simulink model "AttitudeKalman2"  (Simulink 6.6)
settings: Solver=ode4  StartTime=0.0  StopTime=500  FixedStep=SampleT  RelTol=1e-3
InitFcn:
  | clc
  | Taxi_Var
  | failures
  | insInit
values from neighbouring files (symbols this model uses):
  A1 = 0    [Taxi_Var.m]    (also in Taxi_Var_new.m = 0.007)
  Apolar = 0.0899    [Taxi_Var.m]    (also in Taxi_Var_new.m = 0.057)
  APtsamp = 0.005    [failures.m]    (also in piccolo_init.m = 0.05)
  b0 = [0.01 0.01 0.01]    [insInit.m]
  CD0 = 0.0219    [Taxi_Var.m]    (also in Taxi_Var_new.m = 0.022)
  chord = S/span    (= 0.384036716878)    [Taxi_Var.m]    (also in Taxi_Var_new.m = 0.351341681574)
  CL0 = 0.1857    [Taxi_Var.m]    (also in Taxi_Var_new.m = 0.38)
  CLa = 4.6206    [Taxi_Var.m]    (also in Taxi_Var_new.m = 18.5)
  CLa_dot = 1.93    [Taxi_Var.m]    (also in Taxi_Var_new.m = 2.64)
  Clb = -0.0043    [Taxi_Var.m]    (also in Taxi_Var_new.m = -0.06)
  ClDa = 0.1695    [Taxi_Var.m]    (also in Taxi_Var_new.m)
  CLDe = 0.4032    [Taxi_Var.m]    (also in Taxi_Var_new.m = 0.24)
  CLDf = 0.047    [Taxi_Var.m]    (also in Taxi_Var_new.m = 0.4)
  ClDr = 0.0003    [Taxi_Var.m]    (also in Taxi_Var_new.m = 0.055)
  Clp = -0.4425    [Taxi_Var.m]    (also in Taxi_Var_new.m = -0.88)
  CLq = 8.7465    [Taxi_Var.m]    (also in Taxi_Var_new.m = 7.4)
  Clr = 0.0675    [Taxi_Var.m]    (also in Taxi_Var_new.m = 0.04)
  Cm0 = -0.0902    [Taxi_Var.m]    (also in Taxi_Var_new.m = 0.56)
  Cm0_factor = 0.9    [failures.m]
  Cm0_fail = 0    [failures.m]
  Cma = -1.3995    [Taxi_Var.m]    (also in Taxi_Var_new.m = -1.58)
  CmDe = -0.9493    [Taxi_Var.m]    (also in Taxi_Var_new.m = -41)
  CmDf = -.021    (= -0.021)    [Taxi_Var.m]    (also in Taxi_Var_new.m)
  Cnb = 0.0281    [Taxi_Var.m]    (also in Taxi_Var_new.m = 0.73)
  CnDa = -0.0031    [Taxi_Var.m]    (also in Taxi_Var_new.m = -0.032)
  CnDr = -0.0882    [Taxi_Var.m]    (also in Taxi_Var_new.m = 0.19)
  Cnp = -0.0695    [Taxi_Var.m]    (also in Taxi_Var_new.m = -0.1)
  Cnr = -0.1045    [Taxi_Var.m]    (also in Taxi_Var_new.m = -0.23)
  CYb = -0.1999    [Taxi_Var.m]    (also in Taxi_Var_new.m = -0.98)
  CYDr = 0.0192    [Taxi_Var.m]    (also in Taxi_Var_new.m = 0.066)
  da_failamp = 5    [failures.m]
  da_failbias = -da_failamp/2    (= -2.5)    [failures.m]
  da_failper = 90    [failures.m]
  daL_fail = 0    [failures.m]
  daR_fail = 0    [failures.m]
  dr_fail = 0    [failures.m]
  dr_failamp = 2    [failures.m]
  dr_failbias = -dr_failamp/2    (= -1)    [failures.m]
  dr_failper = 70    [failures.m]
  Euler_0 = [0; 0; 45]'*pi/180    [Taxi_Var.m]    (also in Taxi_Var_new.m = [0 0 45]'*pi/180)
  Gw = zeros(6,6)    [insInit.m]
  H = [eye(3,3) zeros(3,3)]    [insInit.m]
  ISA_g = 9.815    [Taxi_Var.m]    (also in Taxi_Var_new.m)
  Ixx = 3.689084    [Taxi_Var.m]    (also in Taxi_Var_new.m = 3.8)
  Iyy = 7.43789    [Taxi_Var.m]    (also in Taxi_Var_new.m = 9.58)
  Izz = 10.22202    [Taxi_Var.m]    (also in Taxi_Var_new.m = 9.68)
  mass = 22.5    [Taxi_Var.m]    (also in Taxi_Var_new.m = 8.16466266)
  MinThK = 0.075    [Taxi_Var.m]    (also in Taxi_Var_new.m = 0.077)
  P0 = diag([.3 .3 .3  .3 0.75 0.75 0.75 ])    [insInit.m]
  Pos_0 = [0; 0; 1000]'    [Taxi_Var.m]    (also in Taxi_Var_new.m = [0 0 500]')
  PQR_0 = [0; 0; 0]'    [Taxi_Var.m]    (also in Taxi_Var_new.m = [ 0 0 0]'*pi/180)
  Rv = rvv^2*eye(3)    [insInit.m]
  SampleT = 0.005    [failures.m]
  span = 2.3368    [Taxi_Var.m]    (also in Taxi_Var_new.m = 2.795)
  tfailure = 20    [failures.m]
  ThK = 2.18    [Taxi_Var.m]    (also in Taxi_Var_new.m = 2.17)
  Vb_0 = [35; 0; 0]'    [Taxi_Var.m]    (also in Taxi_Var_new.m = [35 0 0]')
undefined symbols (not defined in the file or in its folder): clock, DiscIntNeverNeededParam, Earth, q0, Rw, sigbuilder_block, WGS84
libraries: simulink x25, aerolibconvert2 x8, aerolibactuator x6, dspsigops x5, aerolibutil x5, dspmtrx3 x4, aerolibtransform2 x3, aerolibatmos2 x2, aerolibnav x2, dspinverses x1
(part 2 of 2)

== system AttitudeKalman2/Plant Model/Plant/6-DOF EOM/Get Euler Dot ==
  p,q,r : Inport
  Euler : Inport  Port=2
  Mux1 : Mux  Inputs=[3 3]
  Mux2 : Mux  Inputs=3
  phidot : Fcn  Expr=u[1]+u[2]*sin(u[4])*tan(u[5])+u[3]*cos(u[4])*tan(u[5])
  psidot : Fcn  Expr=u[2]*sin(u[4])/cos(u[5])+u[3]*cos(u[4])/cos(u[5])
  thetadot : Fcn  Expr=u[2]*cos(u[4])-u[3]*sin(u[4])
  Euler_dot : Outport
  wires:
  Mux2/1 -> Euler_dot/1
  phidot/1 -> Mux2/1
  thetadot/1 -> Mux2/2
  psidot/1 -> Mux2/3
  Mux1/1 -> thetadot/1, phidot/1, psidot/1
  p,q,r/1 -> Mux1/1
  Euler/1 -> Mux1/2

== system AttitudeKalman2/Plant Model/Plant/6-DOF EOM/RB2LTP ==
  Euler : Inport
  11 : Fcn  Expr=cos(u[3])*cos(u[2])
  12 : Fcn  Expr=sin(u[3])*cos(u[2])
  13 : Fcn  Expr=-sin(u[2])
  21 : Fcn  Expr=cos(u[3])*sin(u[2])*sin(u[1])-sin(u[3])*cos(u[1])
  22 : Fcn  Expr=sin(u[3])*sin(u[2])*sin(u[1])+cos(u[3])*cos(u[1])
  23 : Fcn  Expr=cos(u[2])*sin(u[1])
  31 : Fcn  Expr=cos(u[3])*sin(u[2])*cos(u[1])+sin(u[3])*sin(u[1])
  32 : Fcn  Expr=sin(u[3])*sin(u[2])*cos(u[1])-cos(u[3])*sin(u[1])
  33 : Fcn  Expr=cos(u[2])*cos(u[1])
  Mux2 : Mux  Inputs=9
  Reshape : Reshape  OutputDimensionality=Customize  OutputDimensions=[3,3]
  Rot : Outport
  wires:
  33/1 -> Mux2/9
  32/1 -> Mux2/8
  31/1 -> Mux2/7
  23/1 -> Mux2/6
  22/1 -> Mux2/5
  21/1 -> Mux2/4
  13/1 -> Mux2/3
  12/1 -> Mux2/2
  11/1 -> Mux2/1
  Mux2/1 -> Reshape/1
  Euler/1 -> 11/1, 33/1, 32/1, 31/1, 23/1, 22/1, 21/1, 13/1, 12/1
  Reshape/1 -> Rot/1

== system AttitudeKalman2/Plant Model/Plant/6-DOF EOM/[V1,2,3,W1,2,3] ==
  note: V*dot =Inv(A){[F ; M] - SigmaAV*}
  "[F ; M]" : Inport
  Euler : Inport  Port=2
  V* : Inport  Port=3  PortDimensions=6
  A = [M ; J] : Subsystem
  Acc_meas : Product  Inputs=/*  Multiplication=Matrix(*)  SaturateOnIntegerOverflow=on  InputSameDT=on
  Demux : Demux  Outputs=[3;3]
  Get Grav Force in Body : Subsystem
  Gravitational Acc : Constant  Value=[0 0 -ISA_g]  VectorParams1D=off
  Selector3 : Selector  IndexOptions=Index vector (dialog)  Indices=1:3  OutputSizes=1  InputPortWidth=6
  Sigma : Subsystem
  Sigma*A : Product  Multiplication=Matrix(*)  SaturateOnIntegerOverflow=on  InputSameDT=on
  Sigma*A*V* : Product  Multiplication=Matrix(*)  SaturateOnIntegerOverflow=on  InputSameDT=on
  Sum1 : Sum  Inputs=+-|  SaturateOnIntegerOverflow=on  InputSameDT=on
  Sum2 : Sum  Inputs=++|  SaturateOnIntegerOverflow=on  InputSameDT=on
  Terminator1 : Terminator
  "V*dot " : Product  Inputs=/*  Multiplication=Matrix(*)  SaturateOnIntegerOverflow=on  InputSameDT=on
  "Acc_meas " : Outport
  V*dot : Outport  Port=2
  wires:
  Sum1/1 -> "V*dot "/2
  A = [M ; J]/1(A Matrix) -> Sigma*A/2, "V*dot "/1, Acc_meas/1
  Demux/1 -> Terminator1/1
  Sigma/1(Sigma) -> Sigma*A/1
  "[F ; M]"/1 -> Sum1/1, Acc_meas/2
  Sigma*A*V*/1 -> Sum1/2
  Demux/2 -> Sigma/1(pqr)
  V*/1 -> Sigma*A*V*/2, Demux/1
  "V*dot "/1 -> V*dot/1
  Sigma*A/1 -> Sigma*A*V*/1
  Acc_meas/1 -> Selector3/1
  Gravitational Acc/1 -> Get Grav Force in Body/2(Grav Force)
  Euler/1 -> Get Grav Force in Body/1(Euler)
  Selector3/1 -> Sum2/2
  Get Grav Force in Body/1(Grav Force (Body)) -> Sum2/1
  Sum2/1 -> "Acc_meas "/1

== system AttitudeKalman2/Plant Model/Plant/Engine Model/Get To1 ==
  dt : Inport
  Divide : Product  Inputs=3  OutScaling=2^-10
  Math Function : Math  Operator=pow  SaturateOnIntegerOverflow=on
  Math Function1 : Math  Operator=pow  SaturateOnIntegerOverflow=on
  MaxRPM : Gain  Gain=7200  SaturateOnIntegerOverflow=on
  Min RPM : Constant  Value=2000
  Min Th K : Constant  Value=MinThK
  Prop Diameter (in) : Constant  Value=17
  Prop Diameter (in)1 : Constant  Value=2
  Prop Diameter (in)2 : Constant  Value=4
  Saturation : Saturate  UpperLimit=1.0  LowerLimit=0.2
  Sum : Sum  Inputs=|++
  Sum1 : Sum  Inputs=|++
  TFact : simulink/Math Operations/Slider Gain  SystemSampleTime=-1  low=0  gain=0.2  high=1
  Th K : Gain  Gain=ThK  SaturateOnIntegerOverflow=on
  To Constant : Constant  Value=2.83e-12
  RPM : Outport
  To : Outport  Port=2
  wires:
  Min Th K/1 -> Sum1/2
  Sum1/1 -> MaxRPM/1
  dt/1 -> Saturation/1
  Th K/1 -> Sum1/1
  MaxRPM/1 -> Sum/1
  Min RPM/1 -> Sum/2
  Sum/1 -> RPM/1, Math Function/1
  TFact/1 -> To/1
  Divide/1 -> TFact/1
  To Constant/1 -> Divide/3
  Math Function1/1 -> Divide/2
  Math Function/1 -> Divide/1
  Prop Diameter (in)/1 -> Math Function1/1
  Prop Diameter (in)2/1 -> Math Function1/2
  Prop Diameter (in)1/1 -> Math Function/2
  Saturation/1 -> Th K/1

== system AttitudeKalman2/Plant Model/Plant/Forces and Moments/Alpha/Beta ==
  "Vx, Vy, Vz (Body)" : Inport
  Rho : Inport  Port=2
  Constant : Constant  Value=0.5  VectorParams1D=off
  Math Function : Math  Operator=sqrt  SaturateOnIntegerOverflow=on
  Product : Product  Inputs=5  SaturateOnIntegerOverflow=on
  R2D1 : Gain  Gain=180/pi  SaturateOnIntegerOverflow=on
  R2D2 : Gain  Gain=180/pi  SaturateOnIntegerOverflow=on
  Scope : Scope
      settings: YMin=-2.5  YMax=2  SaveName=ScopeData6
  Scope1 : Scope
      settings: YMin=-1.5  YMax=1.5  SaveName=ScopeData8
  V^2 : Fcn  Expr=(u(1)^2+u(2)^2+u(3)^2)
  "[-15; 15 ]" : Saturate  UpperLimit=15  LowerLimit=-15
  "[-15;15]" : Saturate  UpperLimit=15  LowerLimit=-15
  aoa : Trigonometry  Operator=asin
  beta : Trigonometry  Operator=atan
  sin(aoa) : Fcn  Expr=u(3)/sqrt(u(1)^2+u(3)^2)
  span : Constant  Value=span  VectorParams1D=off
  span1 : Constant  Value=chord  VectorParams1D=off
  tan(beta) : Fcn  Expr=u(2)/sqrt(u(1)^2+u(3)^2)
  "alpha, deg" : Outport
  "beta, deg" : Outport  Port=2
  qS : Outport  Port=3
  Speed : Outport  Port=4
  wires:
  "Vx, Vy, Vz (Body)"/1 -> sin(aoa)/1, tan(beta)/1, V^2/1
  tan(beta)/1 -> beta/1
  beta/1 -> R2D1/1
  V^2/1 -> Product/1, Math Function/1
  Rho/1 -> Product/2
  Constant/1 -> Product/3
  Product/1 -> qS/1
  span/1 -> Product/4
  span1/1 -> Product/5
  R2D1/1 -> "[-15; 15 ]"/1  "beta"
  aoa/1 -> R2D2/1
  R2D2/1 -> "[-15;15]"/1  "aoa"
  sin(aoa)/1 -> aoa/1
  Math Function/1 -> Speed/1
  "[-15;15]"/1 -> "alpha, deg"/1, Scope1/1
  "[-15; 15 ]"/1 -> "beta, deg"/1, Scope/1

== system AttitudeKalman2/Plant Model/Plant/Forces and Moments/Body Frame F & M ==
  "Alpha, deg" : Inport
  "Beta, deg" : Inport  Port=2
  qs : Inport  Port=3
  Airspeed : Inport  Port=4
  "de, deg" : Inport  Port=5
  "dr, deg" : Inport  Port=6
  "df, deg" : Inport  Port=7
  "da_L, deg" : Inport  Port=8
  "da_R, deg" : Inport  Port=9
  p,q,r : Inport  Port=10
  Bus Creator : BusCreator  Inputs=2
  Transfer to body frame : Subsystem
  Wind frame F& M : Subsystem
  F_b : Outport
  M_b : Outport  Port=2
  wires:
  "Alpha, deg"/1 -> Wind frame F& M/1("alpha, deg"), Bus Creator/1
  "Beta, deg"/1 -> Wind frame F& M/2("beta, deg"), Bus Creator/2
  "dr, deg"/1 -> Wind frame F& M/4("dr, deg")
  "da_L, deg"/1 -> Wind frame F& M/9("da_L, deg")
  "de, deg"/1 -> Wind frame F& M/3("de, deg")
  Wind frame F& M/1(F&M wind frame) -> Transfer to body frame/1(Wind frame  F&M)
  Bus Creator/1 -> Transfer to body frame/2("aoa/beta, deg")  "aoa/beta, deg"
  Transfer to body frame/1(F_b) -> F_b/1
  Transfer to body frame/2(M_b) -> M_b/1
  "df, deg"/1 -> Wind frame F& M/5("df, deg")
  qs/1 -> Wind frame F& M/6(qS)
  p,q,r/1 -> Wind frame F& M/7(p,q,r)
  Airspeed/1 -> Wind frame F& M/8(Airpseed)
  "da_R, deg"/1 -> Wind frame F& M/10("da_R, deg")

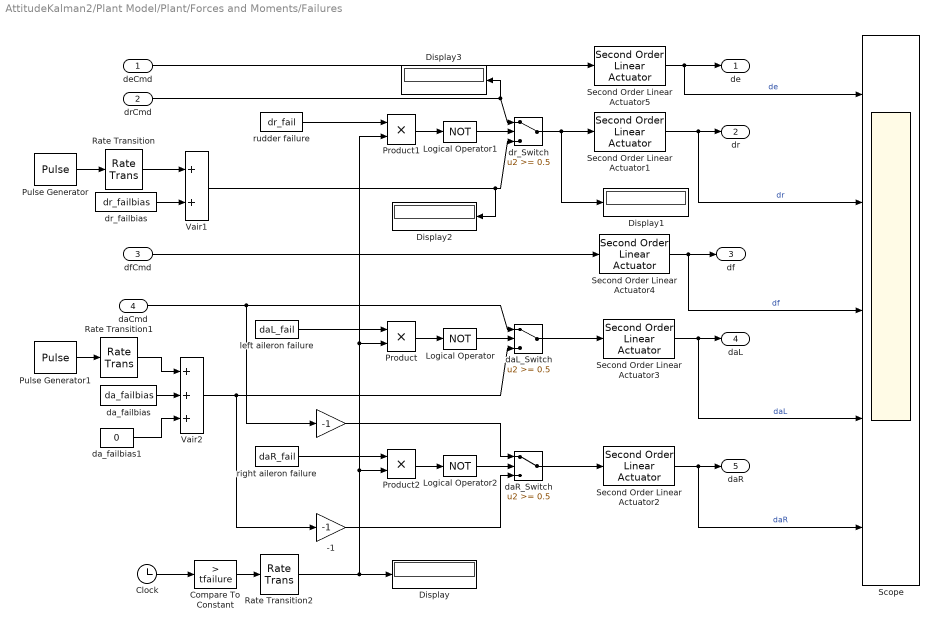
== system AttitudeKalman2/Plant Model/Plant/Forces and Moments/Failures ==
  deCmd : Inport
  drCmd : Inport  Port=2
  dfCmd : Inport  Port=3
  daCmd : Inport  Port=4
  " " : Gain  Gain=-1  SaturateOnIntegerOverflow=on
  "-1 " : Gain  Gain=-1  SaturateOnIntegerOverflow=on
  Clock : Clock
      settings: Decimation=10
  Compare To Constant : simulink/Logic and Bit Operations/Compare To Constant  SystemSampleTime=-1  relop=>  const=tfailure  LogicOutDataTypeMode=uint8  ZeroCross=off
  Display{,1..3} (4 alike) : Display
  Logical Operator : Logic  Operator=NOT  AllPortsSameDT=off  OutDataTypeMode=Boolean
  Logical Operator1 : Logic  Operator=NOT  AllPortsSameDT=off  OutDataTypeMode=Boolean
  Logical Operator2 : Logic  Operator=NOT  AllPortsSameDT=off  OutDataTypeMode=Boolean
  Product : Product  RndMeth=Zero
  Product1 : Product  RndMeth=Zero
  Product2 : Product  RndMeth=Zero
  Pulse Generator : DiscretePulseGenerator  PulseType=Time based  Amplitude=dr_failamp  Period=dr_failper  PulseWidth=50
  Pulse Generator1 : DiscretePulseGenerator  PulseType=Time based  Amplitude=da_failamp  Period=da_failper  PulseWidth=50
  Rate Transition : RateTransition  OutPortSampleTime=APtsamp
  Rate Transition1 : RateTransition  OutPortSampleTime=APtsamp
  Rate Transition2 : RateTransition  OutPortSampleTime=APtsamp
  Scope : Scope  NumInputPorts=5
      settings: YMin=-5~-5~-5~-5~-5  YMax=5~5~5~5~5  SaveName=ScopeData5
  Second Order Linear Actuator{1..5} (5 alike) : aerolibactuator/Second Order Linear Actuator  SystemSampleTime=-1  wn_fin=60  z_fin=0.7  fin_act_0=0
  Vair1 : Sum  SaturateOnIntegerOverflow=on  InputSameDT=on
  Vair2 : Sum  Inputs=+++  SaturateOnIntegerOverflow=on  InputSameDT=on
  daL_Switch : Switch  Threshold=0.5
  daR_Switch : Switch  Threshold=0.5
  da_failbias : Constant  Value=da_failbias  SampleTime=APtsamp
  da_failbias1 : Constant  Value=0  SampleTime=APtsamp
  dr_Switch : Switch  Threshold=0.5
  dr_failbias : Constant  Value=dr_failbias  SampleTime=APtsamp
  left aileron failure : Constant  Value=daL_fail  SampleTime=APtsamp
  right aileron failure : Constant  Value=daR_fail  SampleTime=APtsamp
  rudder failure : Constant  Value=dr_fail  SampleTime=APtsamp
  de : Outport
  dr : Outport  Port=2
  df : Outport  Port=3
  daL : Outport  Port=4
  daR : Outport  Port=5
  wires:
  Pulse Generator/1 -> Rate Transition/1
  dr_failbias/1 -> Vair1/2
  deCmd/1 -> Second Order Linear Actuator5/1
  dr_Switch/1 -> Second Order Linear Actuator1/1, Display1/1
  rudder failure/1 -> Product1/1
  drCmd/1 -> dr_Switch/1, Display3/1
  Vair1/1 -> dr_Switch/3, Display2/1
  dfCmd/1 -> Second Order Linear Actuator4/1
  Pulse Generator1/1 -> Rate Transition1/1
  da_failbias/1 -> Vair2/2
  left aileron failure/1 -> Product/1
  daCmd/1 -> daL_Switch/1, " "/1
  Vair2/1 -> daL_Switch/3, "-1 "/1
  daL_Switch/1 -> Second Order Linear Actuator3/1
  right aileron failure/1 -> Product2/1
  daR_Switch/1 -> Second Order Linear Actuator2/1
  " "/1 -> daR_Switch/1
  "-1 "/1 -> daR_Switch/3
  Second Order Linear Actuator1/1 -> dr/1, Scope/2  "dr"
  Second Order Linear Actuator3/1 -> daL/1, Scope/4  "daL"
  Second Order Linear Actuator2/1 -> daR/1, Scope/5  "daR"
  Second Order Linear Actuator5/1 -> de/1, Scope/1  "de"
  Second Order Linear Actuator4/1 -> df/1, Scope/3  "df"
  Clock/1 -> Compare To Constant/1
  Product/1 -> Logical Operator/1
  Product1/1 -> Logical Operator1/1
  Product2/1 -> Logical Operator2/1
  Compare To Constant/1 -> Rate Transition2/1
  Logical Operator1/1 -> dr_Switch/2
  Logical Operator/1 -> daL_Switch/2
  Logical Operator2/1 -> daR_Switch/2
  da_failbias1/1 -> Vair2/3
  Rate Transition/1 -> Vair1/1
  Rate Transition1/1 -> Vair2/1
  Rate Transition2/1 -> Product2/2, Product/2, Product1/2, Display/1

== system AttitudeKalman2/Plant Model/Plant/Forces and Moments/Get Grav Force in Body ==
  Euler : Inport
  Grav Force : Inport  Port=2
  Math Function : Math  Operator=transpose  SaturateOnIntegerOverflow=on
  Product1 : Product  Multiplication=Matrix(*)  SaturateOnIntegerOverflow=on  InputSameDT=on
  Rb2u : Subsystem
  Reshape : Reshape  OutputDimensionality=Column vector (2-D)
  Grav Force (Body) : Outport
  wires:
  Rb2u/1(DCM) -> Math Function/1
  Euler/1 -> Rb2u/1(phi theta psi)
  Product1/1 -> Grav Force (Body)/1
  Math Function/1 -> Product1/1
  Grav Force/1 -> Reshape/1
  Reshape/1 -> Product1/2

== system AttitudeKalman2/Plant Model/Plant/Forces and Moments/NED(u)2b ==
  V w : Inport
  Euler : Inport  Port=2
  RB2LTP : Subsystem
  RL2B * Vw : Product  Multiplication=Matrix(*)  SaturateOnIntegerOverflow=on  InputSameDT=on
  RLTP2B : Math  Operator=transpose  SaturateOnIntegerOverflow=on
  Reshape1 : Reshape  OutputDimensionality=Row vector (2-D)
  Vb Corr : Outport
  wires:
  RL2B * Vw/1 -> Reshape1/1
  Euler/1 -> RB2LTP/1(Euler)
  RB2LTP/1(RB2L) -> RLTP2B/1
  RLTP2B/1 -> RL2B * Vw/1
  V w/1 -> RL2B * Vw/2
  Reshape1/1 -> Vb Corr/1

== system AttitudeKalman2/Get GPS in LTP/Geod2LTP2/ECEF2LTP (UEN)/From Body to Universal1/Rotation Matrix from Long//Lat ==
  note: Calculate Coefficients of DCM Row-Wise
  long lat : Inport
  11 : Fcn  Expr=cos(u[1])*cos(u[2])
  12 : Fcn  Expr=sin(u[1])*cos(u[2])
  13 : Fcn  Expr=sin(u[2])
  21 : Fcn  Expr=-sin(u[1])
  22 : Fcn  Expr=cos(u[1])
  23 : Fcn  Expr=0
  31 : Fcn  Expr=-sin(u[2])*cos(u[1])
  32 : Fcn  Expr=-sin(u[1])*sin(u[2])
  33 : Fcn  Expr=cos(u[2])
  Mux2 : Mux  Inputs=9
  DCM : Outport  InitialOutput=0
  wires:
  33/1 -> Mux2/9
  23/1 -> Mux2/8
  13/1 -> Mux2/7
  32/1 -> Mux2/6
  22/1 -> Mux2/5
  12/1 -> Mux2/4
  31/1 -> Mux2/3
  21/1 -> Mux2/2
  11/1 -> Mux2/1
  Mux2/1 -> DCM/1
  long lat/1 -> 11/1, 33/1, 23/1, 13/1, 32/1, 22/1, 12/1, 31/1, 21/1

== system AttitudeKalman2/Plant Model/Plant/6-DOF EOM/[V1,2,3,W1,2,3]/A = [M ; J] ==
  Constant1 : Constant  Value=zeros(3,3)
  Constant4 : Constant  Value=0
  Display : Display
  Display1 : Display
  Display2 : Display
  Ixx : Constant  Value=Ixx  VectorParams1D=off
  Iyy : Constant  Value=Iyy  VectorParams1D=off
  Izz : Constant  Value=Izz  VectorParams1D=off
  Matrix Concatenation : Concatenate  Mode=Multidimensional array
  Matrix Concatenation1 : Concatenate  Mode=Multidimensional array
  Matrix Concatenation2 : Concatenate  Mode=Multidimensional array  ConcatenateDimension=2
  Mux : Mux  Inputs=9
  Mux1 : Mux  Inputs=9
  Reshape : Reshape  OutputDimensionality=Customize  OutputDimensions=[3,3]
  Reshape1 : Reshape  OutputDimensionality=Customize  OutputDimensions=[3,3]
  mass : Constant  Value=mass  VectorParams1D=off
  A Matrix : Outport
  wires:
  Constant1/1 -> Matrix Concatenation1/1, Matrix Concatenation/2
  Reshape/1 -> Matrix Concatenation/1
  Reshape1/1 -> Matrix Concatenation1/2
  Matrix Concatenation2/1 -> Display2/1, A Matrix/1
  Matrix Concatenation1/1 -> Display1/1, Matrix Concatenation2/2
  Matrix Concatenation/1 -> Display/1, Matrix Concatenation2/1
  Mux/1 -> Reshape1/1
  Mux1/1 -> Reshape/1
  mass/1 -> Mux1/9, Mux1/5, Mux1/1
  Constant4/1 -> Mux1/2, Mux1/3, Mux1/4, Mux1/6, Mux1/7, Mux1/8, Mux/2, Mux/3, Mux/4, Mux/6, Mux/7, Mux/8
  Iyy/1 -> Mux/5
  Izz/1 -> Mux/9
  Ixx/1 -> Mux/1

== system AttitudeKalman2/Plant Model/Plant/6-DOF EOM/[V1,2,3,W1,2,3]/Get Grav Force in Body ==
  Euler : Inport
  Grav Force : Inport  Port=2
  Math Function : Math  Operator=transpose  SaturateOnIntegerOverflow=on
  Product1 : Product  Multiplication=Matrix(*)  SaturateOnIntegerOverflow=on  InputSameDT=on
  Rb2u : Subsystem
  Reshape : Reshape  OutputDimensionality=Column vector (2-D)
  Grav Force (Body) : Outport
  wires:
  Reshape/1 -> Product1/2
  Grav Force/1 -> Reshape/1
  Math Function/1 -> Product1/1
  Product1/1 -> Grav Force (Body)/1
  Euler/1 -> Rb2u/1(phi theta psi)
  Rb2u/1(DCM) -> Math Function/1

== system AttitudeKalman2/Plant Model/Plant/6-DOF EOM/[V1,2,3,W1,2,3]/Sigma ==
  note: S(pqr)
  pqr : Inport
  Gain : Gain  Gain=[0 0 0;0 0 -1; 0 1 0]  Multiplication=Matrix(K*u)  SaturateOnIntegerOverflow=on
  Gain1 : Gain  Gain=[0 0 1;0 0 0; -1 0 0]  Multiplication=Matrix(K*u)  SaturateOnIntegerOverflow=on
  Gain2 : Gain  Gain="[0 -1 0;1 0 0;  0 0 0]"  Multiplication=Matrix(K*u)  SaturateOnIntegerOverflow=on
  Gain3 : Gain  Gain=0  SaturateOnIntegerOverflow=on
  Math Function : Math  Operator=transpose  SaturateOnIntegerOverflow=on
  Matrix Concatenation : Concatenate  Mode=Multidimensional array  ConcatenateDimension=2
  Matrix Concatenation1 : Concatenate  Mode=Multidimensional array  ConcatenateDimension=2
  Matrix Concatenation2 : Concatenate  Mode=Multidimensional array
  Mux : Mux  Inputs=3
  Reshape : Reshape  OutputDimensionality=Customize  OutputDimensions=[3,3]
  Sigma : Outport
  wires:
  pqr/1 -> Gain1/1, Gain2/1, Gain/1
  Matrix Concatenation2/1 -> Sigma/1
  Matrix Concatenation1/1 -> Matrix Concatenation2/2
  Matrix Concatenation/1 -> Matrix Concatenation2/1
  Gain3/1 -> Matrix Concatenation1/1, Matrix Concatenation/2
  Math Function/1 -> Matrix Concatenation1/2, Matrix Concatenation/1, Gain3/1
  Reshape/1 -> Math Function/1
  Gain2/1 -> Mux/3
  Gain1/1 -> Mux/2
  Gain/1 -> Mux/1
  Mux/1 -> Reshape/1

== system AttitudeKalman2/Plant Model/Plant/Forces and Moments/Body Frame F & M/Transfer to body frame ==
  Wind frame  F&M : Inport
  "aoa/beta, deg" : Inport  Port=2
  D2R : Gain  Gain=pi/180  SaturateOnIntegerOverflow=on
  Forces : Selector  IndexOptions=Index vector (dialog)  Indices=[1 2 3]  OutputSizes=[(-2)]  InputPortWidth=6
  Moments : Selector  IndexOptions=Index vector (dialog)  Indices=[4 5 6]  OutputSizes=[(-2)]  InputPortWidth=6
  Ra2b1 : Subsystem
  Ra2b22 : Subsystem
  Scope : Scope
      settings: YMin=-450  YMax=200  SaveName=ScopeData11
  F_b : Outport
  M_b : Outport  Port=2
  wires:
  Ra2b1/1(body frame) -> F_b/1, Scope/1  "Fb"
  Ra2b22/1(body frame) -> M_b/1  "Mb"
  "aoa/beta, deg"/1 -> D2R/1
  Forces/1 -> Ra2b1/1(wind frame)
  Wind frame  F&M/1 -> Forces/1, Moments/1
  Moments/1 -> Ra2b22/2(wind frame)
  D2R/1 -> Ra2b1/2(aoa/beta), Ra2b22/1(aoa/beta)

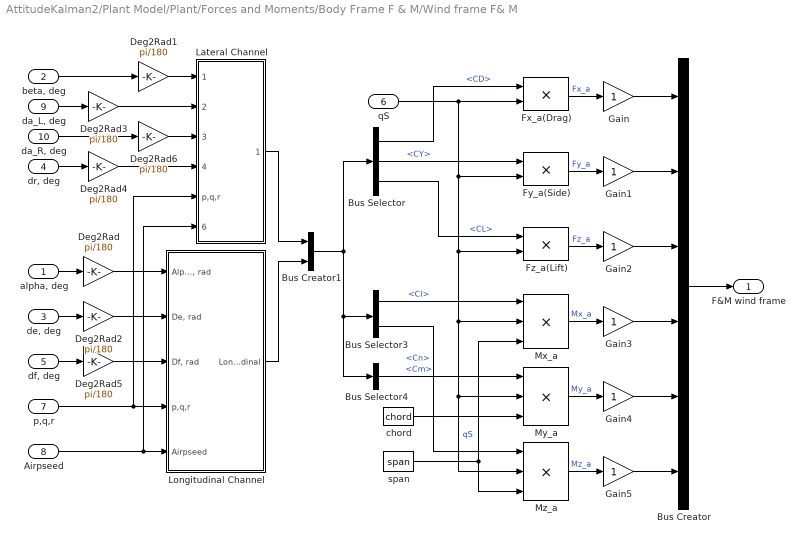
== system AttitudeKalman2/Plant Model/Plant/Forces and Moments/Body Frame F & M/Wind frame F& M ==
  "alpha, deg" : Inport
  "beta, deg" : Inport  Port=2
  "de, deg" : Inport  Port=3
  "dr, deg" : Inport  Port=4
  "df, deg" : Inport  Port=5
  qS : Inport  Port=6
  p,q,r : Inport  Port=7
  Airpseed : Inport  Port=8
  "da_L, deg" : Inport  Port=9
  "da_R, deg" : Inport  Port=10
  Bus Creator : BusCreator  Inputs=6
  Bus Creator1 : BusCreator  Inputs=2
  Bus Selector : BusSelector  OutputSignals=signal2.CD,signal1.CY,signal2.CL
  Bus Selector3 : BusSelector  OutputSignals=signal1.Cl,signal1.Cn
  Bus Selector4 : BusSelector  OutputSignals=signal2.Cm
  Deg2Rad{,1..6} (7 alike) : Gain  Gain=pi/180  SaturateOnIntegerOverflow=on
  Fx_a(Drag) : Product  Inputs=**  SaturateOnIntegerOverflow=on
  Fy_a(Side) : Product  SaturateOnIntegerOverflow=on
  Fz_a(Lift) : Product  SaturateOnIntegerOverflow=on
  Gain{,1..5} (6 alike) : Gain  SaturateOnIntegerOverflow=on
  Lateral Channel : Subsystem
  Longitudinal Channel : Subsystem
  Mx_a : Product  Inputs=3  SaturateOnIntegerOverflow=on
  My_a : Product  Inputs=3  SaturateOnIntegerOverflow=on
  Mz_a : Product  Inputs=3  SaturateOnIntegerOverflow=on
  chord : Constant  Value=chord  VectorParams1D=off
  span : Constant  Value=span  VectorParams1D=off
  F&M wind frame : Outport
  wires:
  Bus Selector/1 -> Fx_a(Drag)/1  "<CD>"
  Fx_a(Drag)/1 -> Gain/1  "Fx_a"
  Fy_a(Side)/1 -> Gain1/1  "Fy_a"
  Fz_a(Lift)/1 -> Gain2/1  "Fz_a"
  Bus Selector3/1 -> Mx_a/1  "<Cl>"
  Mx_a/1 -> Gain3/1  "Mx_a"
  Bus Selector4/1 -> My_a/1  "<Cm>"
  Mz_a/1 -> Gain5/1  "Mz_a"
  qS/1 -> Fx_a(Drag)/2, Fy_a(Side)/2, Fz_a(Lift)/2, Mx_a/2, My_a/2, Mz_a/2  "qS"
  span/1 -> Mx_a/3, Mz_a/3
  chord/1 -> My_a/3
  Bus Selector/2 -> Fy_a(Side)/1  "<CY>"
  Bus Selector/3 -> Fz_a(Lift)/1  "<CL>"
  Bus Selector3/2 -> Mz_a/1  "<Cn>"
  Bus Creator/1 -> F&M wind frame/1
  My_a/1 -> Gain4/1  "My_a"
  Bus Creator1/1 -> Bus Selector/1, Bus Selector3/1, Bus Selector4/1
  Longitudinal Channel/1(Longitudinal) -> Bus Creator1/2
  "alpha, deg"/1 -> Deg2Rad/1
  "beta, deg"/1 -> Deg2Rad1/1
  "de, deg"/1 -> Deg2Rad2/1
  "da_L, deg"/1 -> Deg2Rad3/1
  "dr, deg"/1 -> Deg2Rad4/1
  Deg2Rad1/1 -> Lateral Channel/1("beta, rad")
  Deg2Rad4/1 -> Lateral Channel/4("Dr, rad")
  Deg2Rad/1 -> Longitudinal Channel/1("Alpha, rad")
  Deg2Rad2/1 -> Longitudinal Channel/2("De, rad")
  Gain/1 -> Bus Creator/1
  Gain1/1 -> Bus Creator/2
  Gain2/1 -> Bus Creator/3
  Gain3/1 -> Bus Creator/4
  Gain4/1 -> Bus Creator/5
  Gain5/1 -> Bus Creator/6
  "df, deg"/1 -> Deg2Rad5/1
  Deg2Rad5/1 -> Longitudinal Channel/3("Df, rad")
  Lateral Channel/1(Lateral) -> Bus Creator1/1
  p,q,r/1 -> Lateral Channel/5(p,q,r), Longitudinal Channel/4(p,q,r)
  Airpseed/1 -> Lateral Channel/6(Airspeed), Longitudinal Channel/5(Airpseed)
  Deg2Rad3/1 -> Lateral Channel/2("Da L, rad")
  Deg2Rad6/1 -> Lateral Channel/3("Da R, rad")
  "da_R, deg"/1 -> Deg2Rad6/1

== system AttitudeKalman2/Plant Model/Plant/Forces and Moments/Get Grav Force in Body/Rb2u ==
  phi theta psi : Inport
  11 : Fcn  Expr=cos(u[3])*cos(u[2])
  12 : Fcn  Expr=sin(u[3])*cos(u[2])
  13 : Fcn  Expr=-sin(u[2])
  21 : Fcn  Expr=cos(u[3])*sin(u[2])*sin(u[1])-sin(u[3])*cos(u[1])
  22 : Fcn  Expr=sin(u[3])*sin(u[2])*sin(u[1])+cos(u[3])*cos(u[1])
  23 : Fcn  Expr=cos(u[2])*sin(u[1])
  31 : Fcn  Expr=cos(u[3])*sin(u[2])*cos(u[1])+sin(u[3])*sin(u[1])
  32 : Fcn  Expr=sin(u[3])*sin(u[2])*cos(u[1])-cos(u[3])*sin(u[1])
  33 : Fcn  Expr=cos(u[2])*cos(u[1])
  Mux2 : Mux  Inputs=9
  Reshape : Reshape  OutputDimensionality=Customize  OutputDimensions=[3,3]
  DCM : Outport  InitialOutput=0
  wires:
  Reshape/1 -> DCM/1
  phi theta psi/1 -> 12/1, 13/1, 21/1, 22/1, 23/1, 31/1, 32/1, 33/1, 11/1
  Mux2/1 -> Reshape/1
  11/1 -> Mux2/1
  12/1 -> Mux2/2
  13/1 -> Mux2/3
  21/1 -> Mux2/4
  22/1 -> Mux2/5
  23/1 -> Mux2/6
  31/1 -> Mux2/7
  32/1 -> Mux2/8
  33/1 -> Mux2/9

== system AttitudeKalman2/Plant Model/Plant/Forces and Moments/NED(u)2b/RB2LTP ==
  Euler : Inport
  11 : Fcn  Expr=cos(u[3])*cos(u[2])
  12 : Fcn  Expr=sin(u[3])*cos(u[2])
  13 : Fcn  Expr=-sin(u[2])
  21 : Fcn  Expr=cos(u[3])*sin(u[2])*sin(u[1])-sin(u[3])*cos(u[1])
  22 : Fcn  Expr=sin(u[3])*sin(u[2])*sin(u[1])+cos(u[3])*cos(u[1])
  23 : Fcn  Expr=cos(u[2])*sin(u[1])
  31 : Fcn  Expr=cos(u[3])*sin(u[2])*cos(u[1])+sin(u[3])*sin(u[1])
  32 : Fcn  Expr=sin(u[3])*sin(u[2])*cos(u[1])-cos(u[3])*sin(u[1])
  33 : Fcn  Expr=cos(u[2])*cos(u[1])
  Mux2 : Mux  Inputs=9
  Reshape : Reshape  OutputDimensionality=Customize  OutputDimensions=[3,3]
  RB2L : Outport  InitialOutput=0
  wires:
  33/1 -> Mux2/9
  32/1 -> Mux2/8
  31/1 -> Mux2/7
  23/1 -> Mux2/6
  22/1 -> Mux2/5
  21/1 -> Mux2/4
  13/1 -> Mux2/3
  12/1 -> Mux2/2
  11/1 -> Mux2/1
  Mux2/1 -> Reshape/1
  Euler/1 -> 11/1, 33/1, 32/1, 31/1, 23/1, 22/1, 21/1, 13/1, 12/1
  Reshape/1 -> RB2L/1

== system AttitudeKalman2/Plant Model/Plant/6-DOF EOM/[V1,2,3,W1,2,3]/Get Grav Force in Body/Rb2u ==
  phi theta psi : Inport
  11 : Fcn  Expr=cos(u[3])*cos(u[2])
  12 : Fcn  Expr=sin(u[3])*cos(u[2])
  13 : Fcn  Expr=-sin(u[2])
  21 : Fcn  Expr=cos(u[3])*sin(u[2])*sin(u[1])-sin(u[3])*cos(u[1])
  22 : Fcn  Expr=sin(u[3])*sin(u[2])*sin(u[1])+cos(u[3])*cos(u[1])
  23 : Fcn  Expr=cos(u[2])*sin(u[1])
  31 : Fcn  Expr=cos(u[3])*sin(u[2])*cos(u[1])+sin(u[3])*sin(u[1])
  32 : Fcn  Expr=sin(u[3])*sin(u[2])*cos(u[1])-cos(u[3])*sin(u[1])
  33 : Fcn  Expr=cos(u[2])*cos(u[1])
  Mux2 : Mux  Inputs=9
  Reshape : Reshape  OutputDimensionality=Customize  OutputDimensions=[3,3]
  DCM : Outport  InitialOutput=0
  wires:
  33/1 -> Mux2/9
  32/1 -> Mux2/8
  31/1 -> Mux2/7
  23/1 -> Mux2/6
  22/1 -> Mux2/5
  21/1 -> Mux2/4
  13/1 -> Mux2/3
  12/1 -> Mux2/2
  11/1 -> Mux2/1
  Mux2/1 -> Reshape/1
  phi theta psi/1 -> 11/1, 33/1, 32/1, 31/1, 23/1, 22/1, 21/1, 13/1, 12/1
  Reshape/1 -> DCM/1

== system AttitudeKalman2/Plant Model/Plant/Forces and Moments/Body Frame F & M/Transfer to body frame/Ra2b1 ==
  wind frame : Inport
  aoa/beta : Inport  Port=2
  Product2 : Product  Multiplication=Matrix(*)  SaturateOnIntegerOverflow=on
  RB2W : Subsystem
  RW2B : Math  Operator=transpose  SaturateOnIntegerOverflow=on
  Reshape : Reshape  OutputDimensionality=Column vector (2-D)
  body frame : Outport
  wires:
  RB2W/1(Rw2b) -> RW2B/1
  aoa/beta/1 -> RB2W/1(aoa beta)
  Product2/1 -> body frame/1
  wind frame/1 -> Reshape/1
  Reshape/1 -> Product2/2
  RW2B/1 -> Product2/1

== system AttitudeKalman2/Plant Model/Plant/Forces and Moments/Body Frame F & M/Transfer to body frame/Ra2b22 ==
  aoa/beta : Inport
  wind frame : Inport  Port=2
  Product2 : Product  Multiplication=Matrix(*)  SaturateOnIntegerOverflow=on
  RB2W : Subsystem
  RW2B : Math  Operator=transpose  SaturateOnIntegerOverflow=on
  Reshape : Reshape  OutputDimensionality=Column vector (2-D)
  body frame : Outport
  wires:
  Reshape/1 -> Product2/2
  wind frame/1 -> Reshape/1
  Product2/1 -> body frame/1
  aoa/beta/1 -> RB2W/1(aoa beta)
  RB2W/1(Rw2b) -> RW2B/1
  RW2B/1 -> Product2/1

== system AttitudeKalman2/Plant Model/Plant/Forces and Moments/Body Frame F & M/Wind frame F& M/Lateral Channel ==
  "beta, rad" : Inport
  "Da L, rad" : Inport  Port=2
  "Da R, rad" : Inport  Port=3
  "Dr, rad" : Inport  Port=4
  p,q,r : Inport  Port=5
  Airspeed : Inport  Port=6
  Bus Creator : BusCreator  Inputs=3
  CY : Subsystem
  Cl : Subsystem
  Cn : Subsystem
  Lateral : Outport
  wires:
  Bus Creator/1 -> Lateral/1
  CY/1(CY) -> Bus Creator/1  "CY"
  Cl/1(Cl) -> Bus Creator/2  "Cl"
  Cn/1(Cn) -> Bus Creator/3  "Cn"
  "beta, rad"/1 -> CY/1(beta), Cn/1(beta), Cl/1(beta)
  "Da L, rad"/1 -> Cn/5(Da_L), Cl/5(Da_L)
  "Dr, rad"/1 -> Cn/2(Dr), CY/2(Dr), Cl/2(Dr)
  Airspeed/1 -> Cn/4(Airspeed), Cl/4(Airspeed)
  p,q,r/1 -> Cn/3(p,q,r), Cl/3(p,q,r)
  "Da R, rad"/1 -> Cl/6(Da_R), Cn/6(Da_R)

== system AttitudeKalman2/Plant Model/Plant/Forces and Moments/Body Frame F & M/Wind frame F& M/Longitudinal Channel ==
  "Alpha, rad" : Inport
  "De, rad" : Inport  Port=2
  "Df, rad" : Inport  Port=3
  p,q,r : Inport  Port=4
  Airpseed : Inport  Port=5
  Bus Creator : BusCreator  Inputs=3
  CD : Subsystem
  CL : Subsystem
  Cm : Subsystem
  Display : Display
  Gain : Gain  Gain=-1  SaturateOnIntegerOverflow=on
  Scope : Scope
      settings: SaveName=ScopeData12
  Transfer Fcn : TransferFcn  Numerator=[1 0]  Denominator=[0.1 1]
  Y-down : Gain  Gain=-1  SaturateOnIntegerOverflow=on
  Longitudinal : Outport
  wires:
  "Alpha, rad"/1 -> CL/1(alpha), Cm/1(alpha), Transfer Fcn/1
  CD/1(CD) -> Gain/1
  Gain/1 -> Bus Creator/1  "CD"
  Y-down/1 -> Bus Creator/2  "CL"
  "De, rad"/1 -> CL/3(De), Cm/2(De)
  CL/1(CL) -> Y-down/1, CD/1(CL)
  Cm/1(Cm) -> Bus Creator/3  "Cm"
  Bus Creator/1 -> Longitudinal/1, Scope/1, Display/1
  "Df, rad"/1 -> Cm/3(Df), CL/4(Df)
  p,q,r/1 -> CL/5(p,q,r)
  Airpseed/1 -> CL/6(Airspeed)
  Transfer Fcn/1 -> CL/2(alpha_dot)

== system AttitudeKalman2/Plant Model/Plant/Forces and Moments/Body Frame F & M/Transfer to body frame/Ra2b1/RB2W ==
  aoa beta : Inport
  11 : Fcn  Expr=cos(u[1])*cos(u[2])
  12 : Fcn  Expr=sin(u[2])
  13 : Fcn  Expr=sin(u[1])*cos(u[2])
  21 : Fcn  Expr=-cos(u[1])*sin(u[2])
  22 : Fcn  Expr=cos(u[2])
  23 : Fcn  Expr=-sin(u[1])*sin(u[2])
  31 : Fcn  Expr=-sin(u[1])
  32 : Fcn  Expr=0
  33 : Fcn  Expr=cos(u[1])
  Mux3 : Mux  Inputs=9
  Reshape 9x1->3x3 : Reshape  OutputDimensionality=Customize  OutputDimensions=[3,3]
  Rw2b : Outport  InitialOutput=0
  wires:
  aoa beta/1 -> 11/1, 21/1, 31/1, 12/1, 22/1, 32/1, 13/1, 23/1, 33/1
  Mux3/1 -> Reshape 9x1->3x3/1
  Reshape 9x1->3x3/1 -> Rw2b/1
  11/1 -> Mux3/1
  21/1 -> Mux3/2
  31/1 -> Mux3/3
  12/1 -> Mux3/4
  22/1 -> Mux3/5
  32/1 -> Mux3/6
  13/1 -> Mux3/7
  23/1 -> Mux3/8
  33/1 -> Mux3/9

== system AttitudeKalman2/Plant Model/Plant/Forces and Moments/Body Frame F & M/Transfer to body frame/Ra2b22/RB2W ==
  aoa beta : Inport
  11 : Fcn  Expr=cos(u[1]) * cos(u[2])
  12 : Fcn  Expr=sin(u[2])
  13 : Fcn  Expr=sin(u[1]) * cos(u[2])
  21 : Fcn  Expr=-cos(u[1]) * sin(u[2])
  22 : Fcn  Expr=cos(u[2])
  23 : Fcn  Expr=-sin(u[1]) * sin(u[2])
  31 : Fcn  Expr=-sin(u[1])
  32 : Fcn  Expr=0
  33 : Fcn  Expr=cos(u[1])
  Mux3 : Mux  Inputs=9
  Reshape 9x1->3x3 : Reshape  OutputDimensionality=Customize  OutputDimensions=[3,3]
  Rw2b : Outport  InitialOutput=0
  wires:
  33/1 -> Mux3/9
  23/1 -> Mux3/8
  13/1 -> Mux3/7
  32/1 -> Mux3/6
  22/1 -> Mux3/5
  12/1 -> Mux3/4
  31/1 -> Mux3/3
  21/1 -> Mux3/2
  11/1 -> Mux3/1
  Reshape 9x1->3x3/1 -> Rw2b/1
  Mux3/1 -> Reshape 9x1->3x3/1
  aoa beta/1 -> 33/1, 23/1, 13/1, 32/1, 22/1, 12/1, 31/1, 21/1, 11/1

== system AttitudeKalman2/Plant Model/Plant/Forces and Moments/Body Frame F & M/Wind frame F& M/Lateral Channel/CY ==
  beta : Inport
  Dr : Inport  Port=2
  CYDr : Constant  Value=CYDr
  CYb : Constant  Value=CYb
  Gain1 : Gain  SaturateOnIntegerOverflow=on
  Gain2 : Gain  SaturateOnIntegerOverflow=on
  Product : Product  SaturateOnIntegerOverflow=on
  Product1 : Product  SaturateOnIntegerOverflow=on
  Sum2 : Sum  SaturateOnIntegerOverflow=on
  CY : Outport
  wires:
  CYb/1 -> Product/1
  Product/1 -> Gain1/1
  beta/1 -> Product/2
  Sum2/1 -> CY/1
  Gain1/1 -> Sum2/1
  CYDr/1 -> Product1/1
  Product1/1 -> Gain2/1
  Dr/1 -> Product1/2
  Gain2/1 -> Sum2/2

== system AttitudeKalman2/Plant Model/Plant/Forces and Moments/Body Frame F & M/Wind frame F& M/Lateral Channel/Cl ==
  beta : Inport
  Dr : Inport  Port=2
  p,q,r : Inport  Port=3
  Airspeed : Inport  Port=4
  Da_L : Inport  Port=5
  Da_R : Inport  Port=6
  ClDa : Constant  Value=ClDa
  "ClDa " : Constant  Value=ClDa
  ClDr : Constant  Value=ClDr
  Clb : Constant  Value=Clb
  Gain1 : Gain  SaturateOnIntegerOverflow=on
  Gain2 : Gain  Gain=-1/2  SaturateOnIntegerOverflow=on
  Gain3 : Gain  Gain=1/2  SaturateOnIntegerOverflow=on
  Gain4 : Gain  SaturateOnIntegerOverflow=on
  Product{1..2,4..5} (4 alike) : Product  SaturateOnIntegerOverflow=on
  Sum : Sum  Inputs=+++++  SaturateOnIntegerOverflow=on
  Sum1 : Sum  Inputs=|++|  SaturateOnIntegerOverflow=on
  roll factors : Subsystem
  Cl : Outport
  wires:
  Airspeed/1 -> roll factors/2(Airspeed)
  p,q,r/1 -> roll factors/1(p,q,r)
  roll factors/1(Clp) -> Sum/4
  roll factors/2(Clr) -> Sum/5
  Gain1/1 -> Sum/3
  Gain4/1 -> Sum/1
  Sum/1 -> Cl/1
  Dr/1 -> Product1/2
  Product1/1 -> Gain1/1
  ClDr/1 -> Product1/1
  Da_L/1 -> Product5/2
  Product5/1 -> Gain3/1
  ClDa/1 -> Product5/1
  beta/1 -> Product4/2
  Product4/1 -> Gain4/1
  Clb/1 -> Product4/1
  Gain3/1 -> Sum1/1
  "ClDa "/1 -> Product2/1
  Gain2/1 -> Sum1/2
  Sum1/1 -> Sum/2
  Product2/1 -> Gain2/1
  Da_R/1 -> Product2/2

== system AttitudeKalman2/Plant Model/Plant/Forces and Moments/Body Frame F & M/Wind frame F& M/Lateral Channel/Cn ==
  beta : Inport
  Dr : Inport  Port=2
  p,q,r : Inport  Port=3
  Airspeed : Inport  Port=4
  Da_L : Inport  Port=5
  Da_R : Inport  Port=6
  CnDa : Constant  Value=CnDa
  CnDa1 : Constant  Value=CnDa
  CnDr : Constant  Value=CnDr
  Cnb : Constant  Value=Cnb
  Gain1 : Gain  SaturateOnIntegerOverflow=on
  Gain2 : Gain  Gain=-1/2  SaturateOnIntegerOverflow=on
  Gain3 : Gain  Gain=1/2  SaturateOnIntegerOverflow=on
  Gain4 : Gain  SaturateOnIntegerOverflow=on
  Product{1..2,4..5} (4 alike) : Product  SaturateOnIntegerOverflow=on
  Sum : Sum  Inputs=+++++  SaturateOnIntegerOverflow=on
  Sum1 : Sum  Inputs=|++|  SaturateOnIntegerOverflow=on
  yaw factors : Subsystem
  Cn : Outport
  wires:
  yaw factors/1(Cnp) -> Sum/4
  yaw factors/2(Cnr) -> Sum/5
  Gain1/1 -> Sum/3
  Gain4/1 -> Sum/1
  Sum/1 -> Cn/1
  Dr/1 -> Product1/2
  Product1/1 -> Gain1/1
  CnDr/1 -> Product1/1
  Da_L/1 -> Product5/2
  Product5/1 -> Gain3/1
  CnDa/1 -> Product5/1
  beta/1 -> Product4/2
  Product4/1 -> Gain4/1
  Cnb/1 -> Product4/1
  p,q,r/1 -> yaw factors/1(p,q,r)
  Airspeed/1 -> yaw factors/2(Airspeed)
  Sum1/1 -> Sum/2
  Gain3/1 -> Sum1/1
  Da_R/1 -> Product2/2
  Product2/1 -> Gain2/1
  CnDa1/1 -> Product2/1
  Gain2/1 -> Sum1/2

== system AttitudeKalman2/Plant Model/Plant/Forces and Moments/Body Frame F & M/Wind frame F& M/Longitudinal Channel/CD ==
  CL : Inport
  " " : Gain  Gain=1.25  SaturateOnIntegerOverflow=on
  "  " : Gain  Gain=1.25  SaturateOnIntegerOverflow=on
  Apolar : Constant  Value=A1
  Apolar (A2) : Constant  Value=Apolar
  CD0 : Constant  Value=CD0
  Math Function : Math  Operator=square  SaturateOnIntegerOverflow=on
  Product : Product  SaturateOnIntegerOverflow=on
  Product1 : Product  SaturateOnIntegerOverflow=on
  Sum1 : Sum  Inputs=+++  SaturateOnIntegerOverflow=on
  CD : Outport
  wires:
  Sum1/1 -> CD/1
  CD0/1 -> " "/1
  CL/1 -> Product1/1, Math Function/1
  Apolar (A2)/1 -> "  "/1
  Product/1 -> Sum1/2
  Apolar/1 -> Product1/2
  Product1/1 -> Sum1/3
  Math Function/1 -> Product/2
  " "/1 -> Sum1/1
  "  "/1 -> Product/1

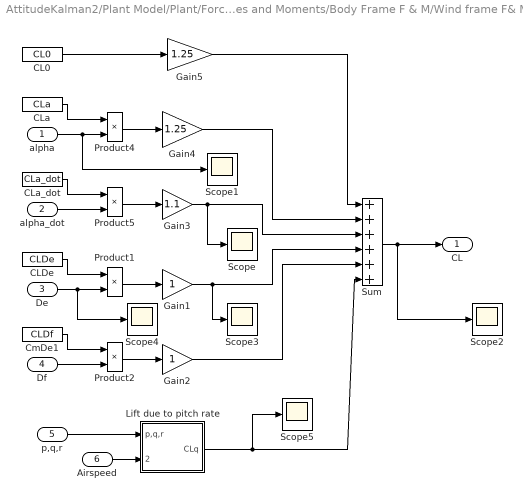
== system AttitudeKalman2/Plant Model/Plant/Forces and Moments/Body Frame F & M/Wind frame F& M/Longitudinal Channel/CL ==
  alpha : Inport
  alpha_dot : Inport  Port=2
  De : Inport  Port=3
  Df : Inport  Port=4
  p,q,r : Inport  Port=5
  Airspeed : Inport  Port=6
  CL0 : Constant  Value=CL0
  CLDe : Constant  Value=CLDe
  CLa : Constant  Value=CLa
  CLa_dot : Constant  Value=CLa_dot
  CmDe1 : Constant  Value=CLDf
  Gain1 : Gain  SaturateOnIntegerOverflow=on
  Gain2 : Gain  SaturateOnIntegerOverflow=on
  Gain3 : Gain  Gain=1.1  SaturateOnIntegerOverflow=on
  Gain4 : Gain  Gain=1.25  SaturateOnIntegerOverflow=on
  Gain5 : Gain  Gain=1.25  SaturateOnIntegerOverflow=on
  Lift due to pitch rate : Subsystem
  Product{1..2,4..5} (4 alike) : Product  SaturateOnIntegerOverflow=on
  Scope{,1..5} (6 alike) : Scope
      Scope settings: YMin=-0.25  YMax=0.075  SaveName=ScopeData7
      Scope1 settings: YMin=-0.45  YMax=0.1  SaveName=ScopeData9
      Scope2 settings: YMin=-0.2  YMax=0.35  SaveName=ScopeData10
      Scope3 settings: YMin=-0.25  YMax=0.075  SaveName=ScopeData15
      Scope4 settings: YMin=-0.25  YMax=0.075  SaveName=ScopeData18
      Scope5 settings: YMin=-0.25  YMax=0.075  SaveName=ScopeData19
  Sum : Sum  Inputs=++++++  SaturateOnIntegerOverflow=on
  CL : Outport
  wires:
  CLa/1 -> Product4/1
  Product4/1 -> Gain4/1
  alpha/1 -> Product4/2, Scope1/1
  CLa_dot/1 -> Product5/1
  Product5/1 -> Gain3/1
  alpha_dot/1 -> Product5/2
  CLDe/1 -> Product1/1
  Product1/1 -> Gain1/1
  De/1 -> Product1/2, Scope4/1
  Sum/1 -> CL/1, Scope2/1
  Df/1 -> Product2/2
  Product2/1 -> Gain2/1
  CmDe1/1 -> Product2/1
  CL0/1 -> Gain5/1
  Gain4/1 -> Sum/2
  Gain3/1 -> Sum/3, Scope/1
  Gain1/1 -> Sum/4, Scope3/1
  Gain2/1 -> Sum/5
  Lift due to pitch rate/1(CLq) -> Sum/6, Scope5/1
  p,q,r/1 -> Lift due to pitch rate/1(p,q,r)
  Airspeed/1 -> Lift due to pitch rate/2(Airspeed)
  Gain5/1 -> Sum/1

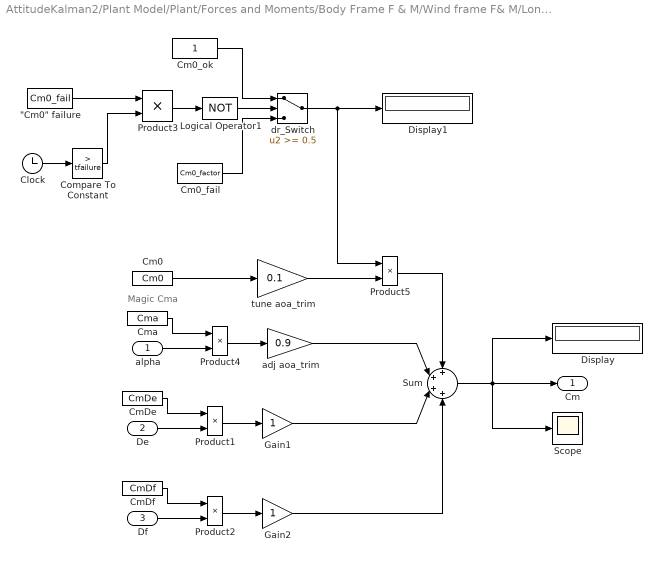
== system AttitudeKalman2/Plant Model/Plant/Forces and Moments/Body Frame F & M/Wind frame F& M/Longitudinal Channel/Cm ==
  note: Magic Cma
  alpha : Inport
  De : Inport  Port=2
  Df : Inport  Port=3
  "\"Cm0\" failure" : Constant  Value=Cm0_fail
  Clock : Clock
      settings: Decimation=10
  Cm0 : Constant  Value=Cm0
  Cm0_fail : Constant  Value=Cm0_factor
  Cm0_ok : Constant
  CmDe : Constant  Value=CmDe
  CmDf : Constant  Value=CmDf
  Cma : Constant  Value=Cma
  Compare To Constant : simulink/Logic and Bit Operations/Compare To Constant  SystemSampleTime=-1  relop=>  const=tfailure  LogicOutDataTypeMode=uint8  ZeroCross=off
  Display : Display
  Display1 : Display
  Gain1 : Gain  SaturateOnIntegerOverflow=on
  Gain2 : Gain  SaturateOnIntegerOverflow=on
  Logical Operator1 : Logic  Operator=NOT  AllPortsSameDT=off  OutDataTypeMode=Boolean
  Product{1..2,4..5} (4 alike) : Product  SaturateOnIntegerOverflow=on
  Product3 : Product  RndMeth=Zero
  Scope : Scope
      settings: SaveName=ScopeData13
  Sum : Sum  Inputs=++++  SaturateOnIntegerOverflow=on
  adj aoa_trim : Gain  Gain=0.9  SaturateOnIntegerOverflow=on
  dr_Switch : Switch  Threshold=0.5
  tune aoa_trim : Gain  Gain=0.1  SaturateOnIntegerOverflow=on
  Cm : Outport
  wires:
  Gain1/1 -> Sum/3
  Cm0/1 -> tune aoa_trim/1
  adj aoa_trim/1 -> Sum/2
  De/1 -> Product1/2
  Product1/1 -> Gain1/1
  CmDe/1 -> Product1/1
  alpha/1 -> Product4/2
  Product4/1 -> adj aoa_trim/1
  Cma/1 -> Product4/1
  Df/1 -> Product2/2
  Product2/1 -> Gain2/1
  CmDf/1 -> Product2/1
  Gain2/1 -> Sum/4
  tune aoa_trim/1 -> Product5/2
  Sum/1 -> Cm/1, Display/1, Scope/1
  Product5/1 -> Sum/1
  "\"Cm0\" failure"/1 -> Product3/1
  Clock/1 -> Compare To Constant/1
  Product3/1 -> Logical Operator1/1
  Compare To Constant/1 -> Product3/2
  Logical Operator1/1 -> dr_Switch/2
  Cm0_fail/1 -> dr_Switch/3
  Cm0_ok/1 -> dr_Switch/1
  dr_Switch/1 -> Product5/1, Display1/1

== system AttitudeKalman2/Plant Model/Plant/Forces and Moments/Body Frame F & M/Wind frame F& M/Lateral Channel/Cl/roll factors ==
  p,q,r : Inport
  Airspeed : Inport  Port=2
  Constant : Constant  Value=Clp
  Constant1 : Constant  Value=Clr
  Get p : Selector  IndexOptions=Index vector (dialog)  Indices=1  OutputSizes=[(-2)]  InputPortWidth=3
  Get r : Selector  IndexOptions=Index vector (dialog)  Indices=3  OutputSizes=[(-2)]  InputPortWidth=3
  Product : Product  SaturateOnIntegerOverflow=on
  Product1 : Product  SaturateOnIntegerOverflow=on
  Slider Gain : simulink/Math Operations/Slider Gain  SystemSampleTime=-1  low=-5  gain=1  high=5
  Slider Gain1 : simulink/Math Operations/Slider Gain  SystemSampleTime=-1  low=-5  gain=1  high=5
  roll rate fact : Subsystem
  yaw rate fact : Subsystem
  Clp : Outport
  Clr : Outport  Port=2
  wires:
  Get r/1 -> yaw rate fact/1(r)
  p,q,r/1 -> Get r/1, Get p/1
  Get p/1 -> roll rate fact/1(p)
  Airspeed/1 -> yaw rate fact/2(Airspeed), roll rate fact/2(Airspeed)
  yaw rate fact/1(Yaw Rate Fac) -> Product1/2
  Slider Gain1/1 -> Product1/1
  roll rate fact/1(Roll Rate Fac) -> Product/2
  Slider Gain/1 -> Product/1
  Product1/1 -> Clr/1
  Product/1 -> Clp/1
  Constant1/1 -> Slider Gain1/1
  Constant/1 -> Slider Gain/1

== system AttitudeKalman2/Plant Model/Plant/Forces and Moments/Body Frame F & M/Wind frame F& M/Lateral Channel/Cn/yaw factors ==
  p,q,r : Inport
  Airspeed : Inport  Port=2
  Constant : Constant  Value=Cnp
  Constant1 : Constant  Value=Cnr
  Get p : Selector  IndexOptions=Index vector (dialog)  Indices=1  OutputSizes=[(-2)]  InputPortWidth=3
  Get r : Selector  IndexOptions=Index vector (dialog)  Indices=3  OutputSizes=[(-2)]  InputPortWidth=3
  Product : Product  SaturateOnIntegerOverflow=on
  Product1 : Product  SaturateOnIntegerOverflow=on
  Slider Gain : simulink/Math Operations/Slider Gain  SystemSampleTime=-1  low=-5  gain=1  high=5
  Slider Gain1 : simulink/Math Operations/Slider Gain  SystemSampleTime=-1  low=-5  gain=1  high=5
  roll rate fact : Subsystem
  yaw rate fact : Subsystem
  Cnp : Outport
  Cnr : Outport  Port=2
  wires:
  Product/1 -> Cnp/1
  Product1/1 -> Cnr/1
  Constant1/1 -> Slider Gain1/1
  Slider Gain1/1 -> Product1/1
  yaw rate fact/1(Yaw Rate Fac) -> Product1/2
  Constant/1 -> Slider Gain/1
  Slider Gain/1 -> Product/1
  roll rate fact/1(Roll Rate Fac) -> Product/2
  Get p/1 -> roll rate fact/1(p)
  p,q,r/1 -> Get p/1, Get r/1
  Get r/1 -> yaw rate fact/1(r)
  Airspeed/1 -> roll rate fact/2(Airspeed), yaw rate fact/2(Airspeed)

== system AttitudeKalman2/Plant Model/Plant/Forces and Moments/Body Frame F & M/Wind frame F& M/Longitudinal Channel/CL/Lift due to pitch rate ==
  p,q,r : Inport
  Airspeed : Inport  Port=2
  Constant : Constant  Value=CLq
  Get q : Selector  IndexOptions=Index vector (dialog)  Indices=2  OutputSizes=[(-2)]  InputPortWidth=3
  Product : Product  SaturateOnIntegerOverflow=on
  pitch rate factor : Subsystem
  CLq : Outport
  wires:
  pitch rate factor/1(Pitch Rate Fac) -> Product/2
  Constant/1 -> Product/1
  Product/1 -> CLq/1
  p,q,r/1 -> Get q/1
  Get q/1 -> pitch rate factor/1(q)
  Airspeed/1 -> pitch rate factor/2(Airspeed)

== system AttitudeKalman2/Plant Model/Plant/Forces and Moments/Body Frame F & M/Wind frame F& M/Lateral Channel/Cl/roll factors/roll rate fact ==
  p : Inport
  Airspeed : Inport  Port=2
  Cmq1 : Constant  Value=.5
  Cmq2 : Constant  Value=span
  Product : Product  Inputs=***/  SaturateOnIntegerOverflow=on
  Roll Rate Fac : Outport
  wires:
  Airspeed/1 -> Product/4
  Cmq2/1 -> Product/3
  Cmq1/1 -> Product/2
  p/1 -> Product/1
  Product/1 -> Roll Rate Fac/1

== system AttitudeKalman2/Plant Model/Plant/Forces and Moments/Body Frame F & M/Wind frame F& M/Lateral Channel/Cl/roll factors/yaw rate fact ==
  r : Inport
  Airspeed : Inport  Port=2
  Cmq1 : Constant  Value=.5
  Cmq2 : Constant  Value=span
  Product : Product  Inputs=***/  SaturateOnIntegerOverflow=on
  Yaw Rate Fac : Outport
  wires:
  Product/1 -> Yaw Rate Fac/1
  Cmq2/1 -> Product/3
  Airspeed/1 -> Product/4
  Cmq1/1 -> Product/2
  r/1 -> Product/1

== system AttitudeKalman2/Plant Model/Plant/Forces and Moments/Body Frame F & M/Wind frame F& M/Lateral Channel/Cn/yaw factors/roll rate fact ==
  p : Inport
  Airspeed : Inport  Port=2
  Cmq1 : Constant  Value=.5
  Cmq2 : Constant  Value=span
  Product : Product  Inputs=***/  SaturateOnIntegerOverflow=on
  Roll Rate Fac : Outport
  wires:
  Product/1 -> Roll Rate Fac/1
  p/1 -> Product/1
  Cmq1/1 -> Product/2
  Cmq2/1 -> Product/3
  Airspeed/1 -> Product/4

== system AttitudeKalman2/Plant Model/Plant/Forces and Moments/Body Frame F & M/Wind frame F& M/Lateral Channel/Cn/yaw factors/yaw rate fact ==
  r : Inport
  Airspeed : Inport  Port=2
  Cmq3 : Constant  Value=.5
  Cmq4 : Constant  Value=span
  Product1 : Product  Inputs=***/  SaturateOnIntegerOverflow=on
  Yaw Rate Fac : Outport
  wires:
  Product1/1 -> Yaw Rate Fac/1
  r/1 -> Product1/1
  Cmq3/1 -> Product1/2
  Cmq4/1 -> Product1/3
  Airspeed/1 -> Product1/4

== system AttitudeKalman2/Plant Model/Plant/Forces and Moments/Body Frame F & M/Wind frame F& M/Longitudinal Channel/CL/Lift due to pitch rate/pitch rate factor ==
  q : Inport
  Airspeed : Inport  Port=2
  Cmq2 : Constant  Value=chord
  Product : Product  Inputs=**/  SaturateOnIntegerOverflow=on
  Pitch Rate Fac : Outport
  wires:
  Product/1 -> Pitch Rate Fac/1
  q/1 -> Product/1
  Airspeed/1 -> Product/3
  Cmq2/1 -> Product/2

== matlab function Kalman Filter/Time Update/Embedded MATLAB Function1 ==
  data: omega input inherited; O output inherited
function O = getOmega(omega)
% This block supports an embeddable subset of the MATLAB language.
% See the help menu for details. 

O=zeros(4,4);
O(1,2:4) = -omega;
O(2:4,1) = transpose(omega);
O(2:4,2:4) = [0 omega(3) -omega(2);...
            -omega(3) 0 omega(1); ...
            omega(2) -omega(1) 0];

== matlab function Kalman Filter/Time Update/Embedded MATLAB Function ==
  data: omega input inherited; F output inherited
function F = getF(omega)
% This block supports an embeddable subset of the MATLAB language.
% See the help menu for details. 

F=zeros(6,6);
F(1:3,4:6) = 0.5*eye(3);
F(1:3,1:3) = [0 omega(3) -omega(2);...
            -omega(3) 0 omega(1); ...
            omega(2) -omega(1) 0];

== matlab function Kalman Filter/Measurement Update/Compute Gb/Embedded MATLAB Function ==
  data: psi input inherited; Cnb output inherited
function Cnb = getCnb(psi)
% This block supports an embeddable subset of the MATLAB language.
% See the help menu for details. 

Cnb=zeros(3,3);
Cnb = [cos(psi) sin(psi) 0; ...
       -sin(psi) cos(psi) 0;
       0 0 1];

== matlab function Kalman Filter/Measurement Update/Compute Gb/Embedded MATLAB Function1 ==
  data: sog input inherited; cog input inherited; Vn output inherited; Ve output inherited
function [Vn,Ve] = getVs(sog, cog)
% This block supports an embeddable subset of the MATLAB language.
% See the help menu for details. 

if (cog<= 90.0)
    Vn = sog*sin(cog);
    Ve = sog*cos(cog);
elseif (cog>90.0 && cog <=180.0)
    Vn = -sog*cos(cog-90);
    Ve = sog*sin(cog-90);
elseif (cog>180.0 && cog<=270.0)
    Vn = -sog*sin(cog-180);
    Ve = -sog*cos(cog-180);
else
    Vn = sog*cos(cog-270);
    Ve = -sog*sin(cog-270);    
end;
